simulink model "simrfV2_qpsk"  (R2020b)
settings: Solver=FixedStepDiscrete  StartTime=0.0  StopTime=1600 * SimPars.SampleTime  RelTol=1e-3  EnableMultiTasking=on
PreLoadFcn:
  | SimPars = simrfV2_qpsk_init();
  | load simrfV2_qpsk_patch_antenna.mat;
values from neighbouring files (symbols this model uses):
  lambda = 0.0045423099697    [simrfV2_qpsk_patch_antenna.mat]    (also in simrfV2_qpsk_patch_array_design.m = ps/F0)
  P_isolated = [-26.1777052768 -19.5496256167 -16.1791035724 -14.0467118928 -12.5793492493 -11.5572548786 -10.8860418126 -10.5241336443 -10.4498816598 -10.6370061743 -11.0230573893 -11.4646926094 ... (2701 elements, 37x73)]    [simrfV2_qpsk_patch_antenna.mat]    (also in simrfV2_qpsk_patch_array_design.m = pattern(p, F0))
undefined symbols (not defined in the file or in its folder): phased, physconst, S
libraries: simrfV2util1 x44, simrfV2elements x40, simrfV2junction1 x28, simrfV2systems x8, commrflib2 x3, commdigbbndpm3 x3, dspsigops x3, dspmathops x3, phasedtxrxlib x3, commutil2 x2, commsequence2 x2, commsync2 x2
(part 2 of 2)

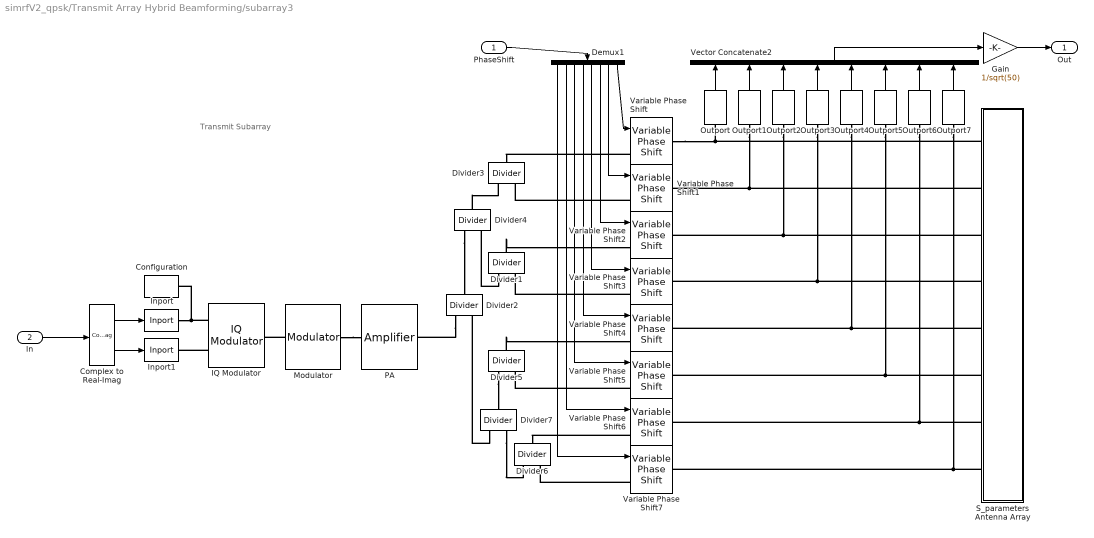
== system simrfV2_qpsk/Transmit Array Hybrid Beamforming/subarray3 ==
  note: Transmit Subarray
  PhaseShift : Inport  OutDataTypeStr=double
  In : Inport  Port=2  OutDataTypeStr=double
      settings: SignalType=complex
  Complex to Real-Imag : ComplexToRealImag
  Configuration : simrfV2util1/Configuration  AutoFreq=off  Tones="[5  66] GHz"  Harmonics=[3 1]  NormalizeCarrierPower=on  SolverType=Auto  UseCCode=on  StepSize=SimPars.SampleTime s  AddNoise=on  defaultRNG=on  Seed=0  Temperature=290.0 K  SolverDelFlag=0  AbsTol=1e-6  RelTol=1e-3  MaxIter=10  ErrorEstimationType=2-norm over all variables  EnableInterpFilter=off  HiddenFIRfilterControllerParam=off  SmallSignalApprox=off  AllSimFreqs=on  SimFreqs=[] Hz  SimFreqsInternal=[]  SamplesPerFrame=SimPars.NumSymsPerFrame * SimPars.SamplesPerSymbol
      settings: SourceProductName=RF Blockset
  Demux1 : Demux  Outputs=8
  Divider{1..7} (7 alike) : simrfV2junction1/Divider  classname=dividers  DataSource=Network-parameters  NumPorts=3  DeviceCirculator=Circulator clockwise  DeviceDivider=Wilkinson power divider  DeviceCoupler=Directional coupler  Paramtype=S-parameters  Sparam=[0 0 1; 1 0 0; 0 1 0]  SparamFreq=1e9 Hz  SparamZ0=50  Phase12=0  Phase33=0  Alpha=0  Coupling=0  Directivity=inf  InsertionLoss=inf  ReturnLoss=inf  InternalGrounding=on  SparamRepresentation=Frequency domain  FitOpt=Share all poles  FitTol=-40
      settings: SourceProductName=RF Blockset
  Gain : Gain  Gain=1/sqrt(50)
  IQ Modulator : simrfV2systems/IQ Modulator  classname=iqmod  Source_linear_gain=Available power gain  linear_gain=8 dB  Poly_Coeffs=[0 1]  LOFreq=5e9 Hz  Zin=50  Zout=50  AddIRFilters=off  AddCSFilter=off  InternalGrounding=on  ForceNextInit=off  NFloor=-168  GainMismatch=0.1 dB  PhaseMismatch=1.2 deg  Isolation=80 dB  AddPhaseNoise=off  PhaseNoiseOffset=1  PhaseNoiseLevel=-Inf  AutoImpulseLengthPN=on  ImpulseLengthPN=1e-10  ImpulseLength_unitPN=s  Source_Poly=Even and odd order  IPType=Output  IP2=21 dBm  IP3=30 dBm  P1dB=inf dBm  Psat=inf dBm  Gcomp=inf dBm  DesignMethodIR=Ideal  ResponseTypeIR=Lowpass  ImplementationIR=LC Tee  ImplementationIdealIR=Constant per carrier  ImplementationRationalIR=Transfer function  UseFilterOrderIR=on  FilterOrderIR=3  PassFreq_lpIR=1  PassFreq_lp_unitIR=GHz  PassFreq_hpIR=2  PassFreq_hp_unitIR=GHz  PassFreq_bpIR=[2 3]  PassFreq_bp_unitIR=GHz  PassFreq_bsIR=[1 4]  PassFreq_bs_unitIR=GHz  PassAttenIR=10*log10(2)  StopFreq_lpIR=2  StopFreq_lp_unitIR=GHz  StopFreq_hpIR=1  StopFreq_hp_unitIR=GHz  StopFreq_bpIR=[1.5 3.5]  StopFreq_bp_unitIR=GHz  StopFreq_bsIR=[2.1 2.9]  StopFreq_bs_unitIR=GHz  StopAttenIR=40  RsrcIR=50  RloadIR=50  AutoImpulseLengthIR=on  ImpulseLengthIR=1e-10  ImpulseLength_unitIR=s  DesignMethodCS=Ideal  ResponseTypeCS=Highpass  ImplementationCS=LC Tee  ImplementationIdealCS=Constant per carrier  ImplementationRationalCS=Transfer function  UseFilterOrderCS=on  FilterOrderCS=3  PassFreq_lpCS=1  PassFreq_lp_unitCS=GHz  PassFreq_hpCS=2  PassFreq_hp_unitCS=GHz  PassFreq_bpCS=[2 3]  PassFreq_bp_unitCS=GHz  PassFreq_bsCS=[1 4]  PassFreq_bs_unitCS=GHz  PassAttenCS=10*log10(2)  StopFreq_lpCS=2  StopFreq_lp_unitCS=GHz  StopFreq_hpCS=1  StopFreq_hp_unitCS=GHz  StopFreq_bpCS=[1.5 3.5]  StopFreq_bp_unitCS=GHz  StopFreq_bsCS=[2.1 2.9]  StopFreq_bs_unitCS=GHz  StopAttenCS=40  RsrcCS=50  RloadCS=50  AutoImpulseLengthCS=on  ImpulseLengthCS=1e-10  ImpulseLength_unitCS=s
      settings: SourceProductName=RF Blockset
  Inport : simrfV2util1/Inport  SimulinkInputSignalType=Power  CarrierFreq=0 Hz  ZS=50  InternalGrounding=on
      settings: SourceProductName=RF Blockset
  Inport1 : simrfV2util1/Inport  SimulinkInputSignalType=Power  CarrierFreq=0 Hz  ZS=50  InternalGrounding=on
      settings: SourceProductName=RF Blockset
  Modulator : simrfV2systems/Modulator  classname=rfmod  Source_linear_gain=Available power gain  linear_gain=-5 dB  Poly_Coeffs=[0 1]  LOFreq=61e9 Hz  Zin=50  Zout=50  AddIRFilter=on  AddCSFilter=on  InternalGrounding=on  ForceNextInit=off  Source_Poly=Even and odd order  IPType=Output  IP2=inf dBm  IP3=inf dBm  P1dB=inf dBm  Psat=inf dBm  Gcomp=inf dBm  NF=6  Isolation=100 dB  AddPhaseNoise=off  PhaseNoiseOffset=1  PhaseNoiseLevel=-Inf  AutoImpulseLengthPN=on  ImpulseLengthPN=1e-10  ImpulseLength_unitPN=s  DesignMethodIR=Ideal  ResponseTypeIR=Lowpass  ImplementationIR=LC Tee  ImplementationIdealIR=Constant per carrier  ImplementationRationalIR=Transfer function  UseFilterOrderIR=on  FilterOrderIR=3  PassFreq_lpIR=10  PassFreq_lp_unitIR=GHz  PassFreq_hpIR=2  PassFreq_hp_unitIR=GHz  PassFreq_bpIR=[2 3]  PassFreq_bp_unitIR=GHz  PassFreq_bsIR=[1 4]  PassFreq_bs_unitIR=GHz  PassAttenIR=10*log10(2)  StopFreq_lpIR=2  StopFreq_lp_unitIR=GHz  StopFreq_hpIR=1  StopFreq_hp_unitIR=GHz  StopFreq_bpIR=[1.5 3.5]  StopFreq_bp_unitIR=GHz  StopFreq_bsIR=[2.1 2.9]  StopFreq_bs_unitIR=GHz  StopAttenIR=40  RsrcIR=50  RloadIR=50  AutoImpulseLengthIR=on  ImpulseLengthIR=1e-10  ImpulseLength_unitIR=s  DesignMethodCS=Ideal  ResponseTypeCS=Highpass  ImplementationCS=LC Tee  ImplementationIdealCS=Constant per carrier  ImplementationRationalCS=Transfer function  UseFilterOrderCS=on  FilterOrderCS=3  PassFreq_lpCS=1  PassFreq_lp_unitCS=GHz  PassFreq_hpCS=60  PassFreq_hp_unitCS=GHz  PassFreq_bpCS=[2 3]  PassFreq_bp_unitCS=GHz  PassFreq_bsCS=[1 4]  PassFreq_bs_unitCS=GHz  PassAttenCS=10*log10(2)  StopFreq_lpCS=2  StopFreq_lp_unitCS=GHz  StopFreq_hpCS=1  StopFreq_hp_unitCS=GHz  StopFreq_bpCS=[1.5 3.5]  StopFreq_bp_unitCS=GHz  StopFreq_bsCS=[2.1 2.9]  StopFreq_bs_unitCS=GHz  StopAttenCS=40  RsrcCS=50  RloadCS=50  AutoImpulseLengthCS=on  ImpulseLengthCS=1e-10  ImpulseLength_unitCS=s
      settings: SourceProductName=RF Blockset
  Outport{,1..7} (8 alike) : simrfV2util1/Outport  SensorType=Ideal voltage  OutputFormat=Complex Baseband  CarrierFreq=SimPars.CarrierFreq Hz  ZL=Inf  InternalGrounding=on  StepSize=1e-6 s  AutoStep=on
      settings: SourceProductName=RF Blockset
  PA : simrfV2elements/Amplifier  classname=amplifier  DataSource=Data file  File=unitygain.s2p  Paramtype=S-parameters  Sparam=[0 0;1 0]  SparamFreq=1e9 Hz  SparamZ0=50  Residues=0  Poles=0  DF={0 0; 1 0}  Source_linear_gain=Available power gain  linear_gain=12 dB  Zin=50  Zout=50  Source_Poly=Odd order  Poly_Coeffs=[0 1]  IPType=Output  IP2=inf dBm  IP3=20 dBm  P1dB=33 dBm  Psat=inf dBm  Gcomp=inf dBm  InternalGrounding=on  SourceFreq=Extracted from data source  PlotFreq=[1e9:1e6:3e9] Hz  PlotType=X-Y plane  YParam1=S(1,1)  YFormat1=Magnitude (decibels)  YParam2=None  YFormat2=Magnitude (decibels)  YOption=Linear  XOption=Linear  SparamRepresentation=Time domain (rationalfit)  FitTol=-40  FitOpt=Fit individually  AutoImpulseLength=on  ImpulseLength=1e-10 s  MagModeling=off  AddNoise=on  NoiseType=Noise figure  NoiseDist=White  NF=3  MinNF=0  Gopt=0  RN=0  CarrierFreq=0 Hz  NoiseAutoImpulseLength=on  NoiseImpulseLength=1e-10 s  SpecifyOpFreq=off  OpFreq=0 Hz
      settings: SourceProductName=RF Blockset
  S_parameters Antenna Array : Subsystem
  Variable Phase Shift{,1..7} (8 alike) : simrfV2elements/Variable Phase Shift  classname=varphase  PhaseShift_unit=deg  SparamZ0=50  InternalGrounding=on
      settings: SourceProductName=RF Blockset
  Vector Concatenate2 : Concatenate  NumInputs=8  Mode=Multidimensional array  ConcatenateDimension=2
  Out : Outport  OutDataTypeStr=double  VectorParamsAs1DForOutWhenUnconnected=off
      settings: SignalType=complex
  wires:
  Outport1/1 -> Vector Concatenate2/2
  Demux1/1 -> Variable Phase Shift7/1
  Demux1/8 -> Variable Phase Shift/1
  Outport6/1 -> Vector Concatenate2/7
  Outport4/1 -> Vector Concatenate2/5
  Complex to Real-Imag/2 -> Inport1/1
  Demux1/7 -> Variable Phase Shift1/1
  Demux1/6 -> Variable Phase Shift2/1
  Demux1/5 -> Variable Phase Shift3/1
  Outport/1 -> Vector Concatenate2/1
  In/1 -> Complex to Real-Imag/1
  Vector Concatenate2/1 -> Gain/1
  Complex to Real-Imag/1 -> Inport/1
  Outport2/1 -> Vector Concatenate2/3
  PhaseShift/1 -> Demux1/1
  Outport5/1 -> Vector Concatenate2/6
  Outport3/1 -> Vector Concatenate2/4
  Demux1/2 -> Variable Phase Shift6/1
  Demux1/3 -> Variable Phase Shift5/1
  Outport7/1 -> Vector Concatenate2/8
  Demux1/4 -> Variable Phase Shift4/1
  Gain/1 -> Out/1
  connections:
  Variable Phase Shift/LConn1 -- Divider3/RConn1
  Outport1/LConn1 -- S_parameters Antenna Array/RConn2 -- Variable Phase Shift1/RConn1
  Divider2/LConn1 -- PA/RConn1
  Outport3/LConn1 -- S_parameters Antenna Array/RConn4 -- Variable Phase Shift3/RConn1
  IQ Modulator/LConn2 -- Inport1/RConn1
  Outport7/LConn1 -- S_parameters Antenna Array/RConn8 -- Variable Phase Shift7/RConn1
  Variable Phase Shift7/LConn1 -- Divider6/LConn2
  Inport/RConn1 -- IQ Modulator/LConn1 -- Configuration/LConn1
  Variable Phase Shift3/LConn1 -- Divider1/LConn2
  Variable Phase Shift/RConn1 -- S_parameters Antenna Array/RConn1 -- Outport/LConn1
  Modulator/RConn1 -- PA/LConn1
  Outport2/LConn1 -- S_parameters Antenna Array/RConn3 -- Variable Phase Shift2/RConn1
  Variable Phase Shift5/LConn1 -- Divider5/LConn2
  Outport6/LConn1 -- S_parameters Antenna Array/RConn7 -- Variable Phase Shift6/RConn1
  Outport5/LConn1 -- S_parameters Antenna Array/RConn6 -- Variable Phase Shift5/RConn1
  Variable Phase Shift6/LConn1 -- Divider6/RConn1
  Divider5/RConn1 -- Variable Phase Shift4/LConn1
  Divider1/RConn1 -- Variable Phase Shift2/LConn1
  Divider4/LConn1 -- Divider2/RConn1
  Divider4/RConn1 -- Divider3/LConn1
  Divider1/LConn1 -- Divider4/LConn2
  Divider5/LConn1 -- Divider7/RConn1
  Divider7/LConn2 -- Divider6/LConn1
  Divider7/LConn1 -- Divider2/LConn2
  Variable Phase Shift1/LConn1 -- Divider3/LConn2
  Modulator/LConn1 -- IQ Modulator/RConn1
  Outport4/LConn1 -- S_parameters Antenna Array/RConn5 -- Variable Phase Shift4/RConn1

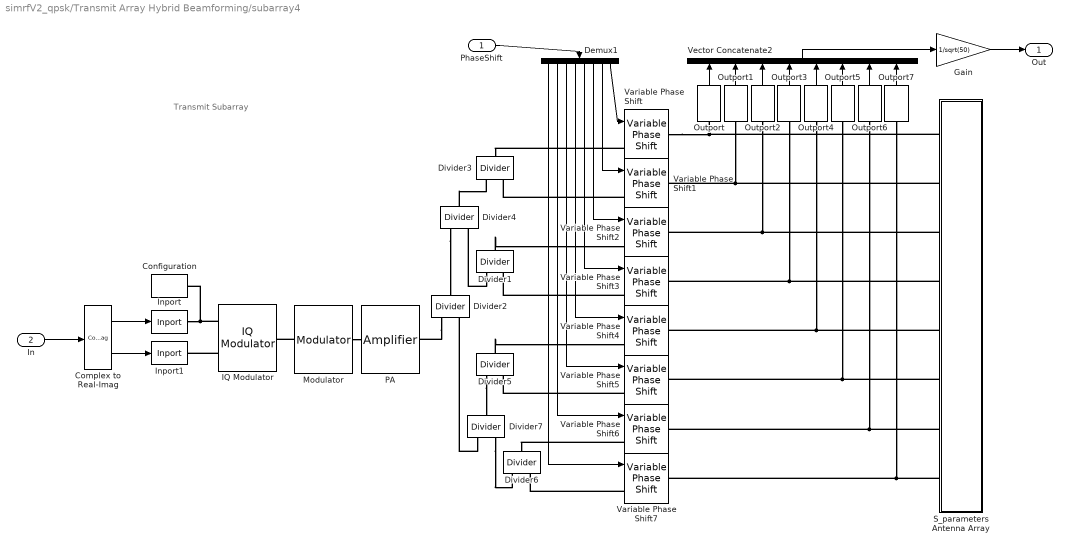
== system simrfV2_qpsk/Transmit Array Hybrid Beamforming/subarray4 ==
  note: Transmit Subarray
  PhaseShift : Inport  OutDataTypeStr=double
  In : Inport  Port=2  OutDataTypeStr=double
      settings: SignalType=complex
  Complex to Real-Imag : ComplexToRealImag
  Configuration : simrfV2util1/Configuration  AutoFreq=off  Tones="[5  66] GHz"  Harmonics=[3 1]  NormalizeCarrierPower=on  SolverType=Auto  UseCCode=on  StepSize=SimPars.SampleTime s  AddNoise=on  defaultRNG=on  Seed=0  Temperature=290.0 K  SolverDelFlag=0  AbsTol=1e-6  RelTol=1e-3  MaxIter=10  ErrorEstimationType=2-norm over all variables  EnableInterpFilter=off  HiddenFIRfilterControllerParam=off  SmallSignalApprox=off  AllSimFreqs=on  SimFreqs=[] Hz  SimFreqsInternal=[]  SamplesPerFrame=SimPars.NumSymsPerFrame * SimPars.SamplesPerSymbol
      settings: SourceProductName=RF Blockset
  Demux1 : Demux  Outputs=8
  Divider{1..7} (7 alike) : simrfV2junction1/Divider  classname=dividers  DataSource=Network-parameters  NumPorts=3  DeviceCirculator=Circulator clockwise  DeviceDivider=Wilkinson power divider  DeviceCoupler=Directional coupler  Paramtype=S-parameters  Sparam=[0 0 1; 1 0 0; 0 1 0]  SparamFreq=1e9 Hz  SparamZ0=50  Phase12=0  Phase33=0  Alpha=0  Coupling=0  Directivity=inf  InsertionLoss=inf  ReturnLoss=inf  InternalGrounding=on  SparamRepresentation=Frequency domain  FitOpt=Share all poles  FitTol=-40
      settings: SourceProductName=RF Blockset
  Gain : Gain  Gain=1/sqrt(50)
  IQ Modulator : simrfV2systems/IQ Modulator  classname=iqmod  Source_linear_gain=Available power gain  linear_gain=8 dB  Poly_Coeffs=[0 1]  LOFreq=5e9 Hz  Zin=50  Zout=50  AddIRFilters=off  AddCSFilter=off  InternalGrounding=on  ForceNextInit=off  NFloor=-168  GainMismatch=0.1 dB  PhaseMismatch=1.2 deg  Isolation=80 dB  AddPhaseNoise=off  PhaseNoiseOffset=1  PhaseNoiseLevel=-Inf  AutoImpulseLengthPN=on  ImpulseLengthPN=1e-10  ImpulseLength_unitPN=s  Source_Poly=Even and odd order  IPType=Output  IP2=21 dBm  IP3=30 dBm  P1dB=inf dBm  Psat=inf dBm  Gcomp=inf dBm  DesignMethodIR=Ideal  ResponseTypeIR=Lowpass  ImplementationIR=LC Tee  ImplementationIdealIR=Constant per carrier  ImplementationRationalIR=Transfer function  UseFilterOrderIR=on  FilterOrderIR=3  PassFreq_lpIR=1  PassFreq_lp_unitIR=GHz  PassFreq_hpIR=2  PassFreq_hp_unitIR=GHz  PassFreq_bpIR=[2 3]  PassFreq_bp_unitIR=GHz  PassFreq_bsIR=[1 4]  PassFreq_bs_unitIR=GHz  PassAttenIR=10*log10(2)  StopFreq_lpIR=2  StopFreq_lp_unitIR=GHz  StopFreq_hpIR=1  StopFreq_hp_unitIR=GHz  StopFreq_bpIR=[1.5 3.5]  StopFreq_bp_unitIR=GHz  StopFreq_bsIR=[2.1 2.9]  StopFreq_bs_unitIR=GHz  StopAttenIR=40  RsrcIR=50  RloadIR=50  AutoImpulseLengthIR=on  ImpulseLengthIR=1e-10  ImpulseLength_unitIR=s  DesignMethodCS=Ideal  ResponseTypeCS=Highpass  ImplementationCS=LC Tee  ImplementationIdealCS=Constant per carrier  ImplementationRationalCS=Transfer function  UseFilterOrderCS=on  FilterOrderCS=3  PassFreq_lpCS=1  PassFreq_lp_unitCS=GHz  PassFreq_hpCS=2  PassFreq_hp_unitCS=GHz  PassFreq_bpCS=[2 3]  PassFreq_bp_unitCS=GHz  PassFreq_bsCS=[1 4]  PassFreq_bs_unitCS=GHz  PassAttenCS=10*log10(2)  StopFreq_lpCS=2  StopFreq_lp_unitCS=GHz  StopFreq_hpCS=1  StopFreq_hp_unitCS=GHz  StopFreq_bpCS=[1.5 3.5]  StopFreq_bp_unitCS=GHz  StopFreq_bsCS=[2.1 2.9]  StopFreq_bs_unitCS=GHz  StopAttenCS=40  RsrcCS=50  RloadCS=50  AutoImpulseLengthCS=on  ImpulseLengthCS=1e-10  ImpulseLength_unitCS=s
      settings: SourceProductName=RF Blockset
  Inport : simrfV2util1/Inport  SimulinkInputSignalType=Power  CarrierFreq=0 Hz  ZS=50  InternalGrounding=on
      settings: SourceProductName=RF Blockset
  Inport1 : simrfV2util1/Inport  SimulinkInputSignalType=Power  CarrierFreq=0 Hz  ZS=50  InternalGrounding=on
      settings: SourceProductName=RF Blockset
  Modulator : simrfV2systems/Modulator  classname=rfmod  Source_linear_gain=Available power gain  linear_gain=-5 dB  Poly_Coeffs=[0 1]  LOFreq=61e9 Hz  Zin=50  Zout=50  AddIRFilter=on  AddCSFilter=on  InternalGrounding=on  ForceNextInit=off  Source_Poly=Even and odd order  IPType=Output  IP2=inf dBm  IP3=inf dBm  P1dB=inf dBm  Psat=inf dBm  Gcomp=inf dBm  NF=6  Isolation=100 dB  AddPhaseNoise=off  PhaseNoiseOffset=1  PhaseNoiseLevel=-Inf  AutoImpulseLengthPN=on  ImpulseLengthPN=1e-10  ImpulseLength_unitPN=s  DesignMethodIR=Ideal  ResponseTypeIR=Lowpass  ImplementationIR=LC Tee  ImplementationIdealIR=Constant per carrier  ImplementationRationalIR=Transfer function  UseFilterOrderIR=on  FilterOrderIR=3  PassFreq_lpIR=10  PassFreq_lp_unitIR=GHz  PassFreq_hpIR=2  PassFreq_hp_unitIR=GHz  PassFreq_bpIR=[2 3]  PassFreq_bp_unitIR=GHz  PassFreq_bsIR=[1 4]  PassFreq_bs_unitIR=GHz  PassAttenIR=10*log10(2)  StopFreq_lpIR=2  StopFreq_lp_unitIR=GHz  StopFreq_hpIR=1  StopFreq_hp_unitIR=GHz  StopFreq_bpIR=[1.5 3.5]  StopFreq_bp_unitIR=GHz  StopFreq_bsIR=[2.1 2.9]  StopFreq_bs_unitIR=GHz  StopAttenIR=40  RsrcIR=50  RloadIR=50  AutoImpulseLengthIR=on  ImpulseLengthIR=1e-10  ImpulseLength_unitIR=s  DesignMethodCS=Ideal  ResponseTypeCS=Highpass  ImplementationCS=LC Tee  ImplementationIdealCS=Constant per carrier  ImplementationRationalCS=Transfer function  UseFilterOrderCS=on  FilterOrderCS=3  PassFreq_lpCS=1  PassFreq_lp_unitCS=GHz  PassFreq_hpCS=60  PassFreq_hp_unitCS=GHz  PassFreq_bpCS=[2 3]  PassFreq_bp_unitCS=GHz  PassFreq_bsCS=[1 4]  PassFreq_bs_unitCS=GHz  PassAttenCS=10*log10(2)  StopFreq_lpCS=2  StopFreq_lp_unitCS=GHz  StopFreq_hpCS=1  StopFreq_hp_unitCS=GHz  StopFreq_bpCS=[1.5 3.5]  StopFreq_bp_unitCS=GHz  StopFreq_bsCS=[2.1 2.9]  StopFreq_bs_unitCS=GHz  StopAttenCS=40  RsrcCS=50  RloadCS=50  AutoImpulseLengthCS=on  ImpulseLengthCS=1e-10  ImpulseLength_unitCS=s
      settings: SourceProductName=RF Blockset
  Outport{,1..7} (8 alike) : simrfV2util1/Outport  SensorType=Ideal voltage  OutputFormat=Complex Baseband  CarrierFreq=SimPars.CarrierFreq Hz  ZL=Inf  InternalGrounding=on  StepSize=1e-6 s  AutoStep=on
      settings: SourceProductName=RF Blockset
  PA : simrfV2elements/Amplifier  classname=amplifier  DataSource=Data file  File=unitygain.s2p  Paramtype=S-parameters  Sparam=[0 0;1 0]  SparamFreq=1e9 Hz  SparamZ0=50  Residues=0  Poles=0  DF={0 0; 1 0}  Source_linear_gain=Available power gain  linear_gain=12 dB  Zin=50  Zout=50  Source_Poly=Odd order  Poly_Coeffs=[0 1]  IPType=Output  IP2=inf dBm  IP3=20 dBm  P1dB=33 dBm  Psat=inf dBm  Gcomp=inf dBm  InternalGrounding=on  SourceFreq=Extracted from data source  PlotFreq=[1e9:1e6:3e9] Hz  PlotType=X-Y plane  YParam1=S(1,1)  YFormat1=Magnitude (decibels)  YParam2=None  YFormat2=Magnitude (decibels)  YOption=Linear  XOption=Linear  SparamRepresentation=Time domain (rationalfit)  FitTol=-40  FitOpt=Fit individually  AutoImpulseLength=on  ImpulseLength=1e-10 s  MagModeling=off  AddNoise=on  NoiseType=Noise figure  NoiseDist=White  NF=3  MinNF=0  Gopt=0  RN=0  CarrierFreq=0 Hz  NoiseAutoImpulseLength=on  NoiseImpulseLength=1e-10 s  SpecifyOpFreq=off  OpFreq=0 Hz
      settings: SourceProductName=RF Blockset
  S_parameters Antenna Array : Subsystem
  Variable Phase Shift{,1..7} (8 alike) : simrfV2elements/Variable Phase Shift  classname=varphase  PhaseShift_unit=deg  SparamZ0=50  InternalGrounding=on
      settings: SourceProductName=RF Blockset
  Vector Concatenate2 : Concatenate  NumInputs=8  Mode=Multidimensional array  ConcatenateDimension=2
  Out : Outport  OutDataTypeStr=double  VectorParamsAs1DForOutWhenUnconnected=off
      settings: SignalType=complex
  wires:
  Outport1/1 -> Vector Concatenate2/2
  Demux1/1 -> Variable Phase Shift7/1
  Demux1/8 -> Variable Phase Shift/1
  Outport6/1 -> Vector Concatenate2/7
  Outport4/1 -> Vector Concatenate2/5
  Complex to Real-Imag/2 -> Inport1/1
  Demux1/7 -> Variable Phase Shift1/1
  Demux1/6 -> Variable Phase Shift2/1
  Demux1/5 -> Variable Phase Shift3/1
  Outport/1 -> Vector Concatenate2/1
  In/1 -> Complex to Real-Imag/1
  Vector Concatenate2/1 -> Gain/1
  Complex to Real-Imag/1 -> Inport/1
  Outport2/1 -> Vector Concatenate2/3
  PhaseShift/1 -> Demux1/1
  Outport5/1 -> Vector Concatenate2/6
  Outport3/1 -> Vector Concatenate2/4
  Demux1/2 -> Variable Phase Shift6/1
  Demux1/3 -> Variable Phase Shift5/1
  Outport7/1 -> Vector Concatenate2/8
  Demux1/4 -> Variable Phase Shift4/1
  Gain/1 -> Out/1
  connections:
  Variable Phase Shift/LConn1 -- Divider3/RConn1
  Outport1/LConn1 -- S_parameters Antenna Array/RConn2 -- Variable Phase Shift1/RConn1
  Divider2/LConn1 -- PA/RConn1
  Outport3/LConn1 -- S_parameters Antenna Array/RConn4 -- Variable Phase Shift3/RConn1
  IQ Modulator/LConn2 -- Inport1/RConn1
  Outport7/LConn1 -- S_parameters Antenna Array/RConn8 -- Variable Phase Shift7/RConn1
  Variable Phase Shift7/LConn1 -- Divider6/LConn2
  Inport/RConn1 -- IQ Modulator/LConn1 -- Configuration/LConn1
  Variable Phase Shift3/LConn1 -- Divider1/LConn2
  Variable Phase Shift/RConn1 -- S_parameters Antenna Array/RConn1 -- Outport/LConn1
  Modulator/RConn1 -- PA/LConn1
  Outport2/LConn1 -- S_parameters Antenna Array/RConn3 -- Variable Phase Shift2/RConn1
  Variable Phase Shift5/LConn1 -- Divider5/LConn2
  Outport6/LConn1 -- S_parameters Antenna Array/RConn7 -- Variable Phase Shift6/RConn1
  Outport5/LConn1 -- S_parameters Antenna Array/RConn6 -- Variable Phase Shift5/RConn1
  Variable Phase Shift6/LConn1 -- Divider6/RConn1
  Divider5/RConn1 -- Variable Phase Shift4/LConn1
  Divider1/RConn1 -- Variable Phase Shift2/LConn1
  Divider4/LConn1 -- Divider2/RConn1
  Divider4/RConn1 -- Divider3/LConn1
  Divider1/LConn1 -- Divider4/LConn2
  Divider5/LConn1 -- Divider7/RConn1
  Divider7/LConn2 -- Divider6/LConn1
  Divider7/LConn1 -- Divider2/LConn2
  Variable Phase Shift1/LConn1 -- Divider3/LConn2
  Modulator/LConn1 -- IQ Modulator/RConn1
  Outport4/LConn1 -- S_parameters Antenna Array/RConn5 -- Variable Phase Shift4/RConn1

== system simrfV2_qpsk/QPSK Receiver/Data Decoding/Barker Code Symbol Generation  ==
  note: Regenerate a QPSK-modulated unipolar Barker code sequence
      | to be compared with the received data
  Constant Barker Code : Constant  Value=SimPars.BarkerCode > 0  VectorParams1D=off  OutDataTypeStr=double
  QPSK Modulator Baseband : commdigbbndpm3/QPSK Modulator Baseband  InType=Bit  Enc=Gray  Ph=pi/4  outDtype=double  outWordLen=16  outUDDataType=sfix(16)  outFracLenMode=Best precision  outFracLen=15  outDataTypeStr=double  outLastDataTypeStr=double
      settings: SourceProductName=Communications Toolbox
  Repeat : dspsigops/Repeat  N=2  InputProcessing=Columns as channels (frame based)  RateOptions=Enforce single-rate processing  ic=0  mode=Unused parameter value
      settings: SourceProductName=DSP System Toolbox
  Out : Outport  VectorParamsAs1DForOutWhenUnconnected=off
  wires:
  Constant Barker Code/1 -> Repeat/1
  Repeat/1 -> QPSK Modulator Baseband/1
  QPSK Modulator Baseband/1 -> Out/1

== system simrfV2_qpsk/QPSK Receiver/Data Decoding/Descrambling ==
  In : Inport
  Descrambler1 : commsequence2/Descrambler  M=2  poly=[1 1 1 0 1]  iniStaSource=Dialog Parameter  ini_sta=[0 0 0 0]  resetViaPort=off
      settings: SourceProductName=Communications Toolbox
  Selector1 : Selector  IndexOptions=Index vector (dialog)  Indices=[2*SimPars.BarkerLength+1:SimPars.NumBitsPerFrame]  OutputSizes=1
  Selector2 : Selector  IndexOptions=Index vector (dialog)  Indices=[1:SimPars.NumMsgBits]  OutputSizes=1
  Out : Outport  VectorParamsAs1DForOutWhenUnconnected=off
  wires:
  In/1 -> Selector1/1
  Selector1/1 -> Descrambler1/1
  Descrambler1/1 -> Selector2/1
  Selector2/1 -> Out/1

== system simrfV2_qpsk/QPSK Receiver/Data Decoding/Phase Ambiguity Correction & Demodulation ==
  note: Phase Ambiguity Resolution
      | and Demodulation
  Phase : Inport
  Data : Inport  Port=2
  Complex Phase Shift : commutil2/Complex Phase Shift
      settings: SourceProductName=Communications Toolbox
  Demodulator Input : ConstellationDiagram
  Gain : Gain  Gain=-1  OutDataTypeStr=Inherit: Same as input
  QPSK Demodulator Baseband : commdigbbndpm3/QPSK Demodulator Baseband  OutType=Bit  DecType=Hard decision  VarSource=Dialog  Variance=1  Dec=Gray  Ph=pi/4  outDtype1=Inherit via internal rule  outDtype2=Inherit via internal rule  derotateFactorWordLen=16  derotateFactorDataTypeStr=Inherit: Same word length as input  derotateFactorLastDataTypeStr=Inherit: Same word length as input
      settings: SourceProductName=Communications Toolbox
  Out : Outport  VectorParamsAs1DForOutWhenUnconnected=off
  wires:
  Phase/1 -> Gain/1
  Complex Phase Shift/1 -> Demodulator Input/1, QPSK Demodulator Baseband/1
  QPSK Demodulator Baseband/1 -> Out/1
  Gain/1 -> Complex Phase Shift/2
  Data/1 -> Complex Phase Shift/1

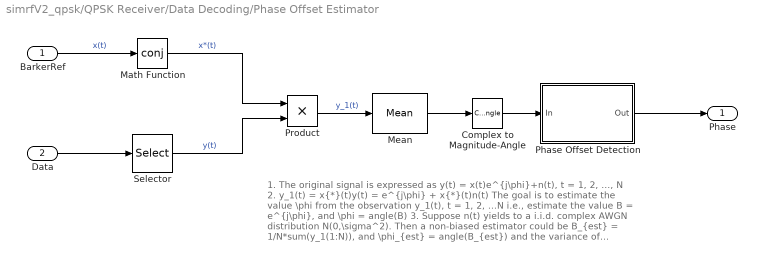
== system simrfV2_qpsk/QPSK Receiver/Data Decoding/Phase Offset Estimator ==
  note: 1. The original signal is expressed as y(t) = x(t)e^{j\phi}+n(t), t = 1, 2, ..., N
      | 2. y_1(t) = x{*}(t)y(t) = e^{j\phi} + x{*}(t)n(t)
      | The goal is to estimate the value \phi from the observation y_1(t), t = 1, 2, ...N
      | i.e., estimate the value B = e^{j\phi}, and \phi = angle(B)
      | 3. Suppose n(t) yields to a i.i.d. complex AWGN distribution N(0,\sigma^2).
      | Then a non-biased estimator could be
      | B_{est} = 1/N*sum(y_1(1:N)), and \phi_{est} = angle(B_{est})
      | and the variance of B_{est} is \sigma^2/N
  BarkerRef : Inport
  Data : Inport  Port=2
  Complex to Magnitude-Angle : ComplexToMagnitudeAngle  Output=Angle
  Math Function : Math  Operator=conj  SignedPower=on  SaturateOnIntegerOverflow=on
  Mean : dspstat3/Mean  run=off  InputProcessing=Columns as channels (frame based)  reset_popup=None  directionMode=Each column  dimension=1  roiEnable=off  roiType=Rectangles  roiPortion=Entire ROI  roiOutput=Individual statistics for each ROI  roiFlag=off  roundingMode=Floor  overflowMode=off  outputDataTypeStr=Inherit: Same as accumulator  outputMin=[]  outputMax=[]  outputLastDataTypeStr=Inherit: Same as accumulator
  Phase Offset Detection : MATLAB Function  TreatAsAtomicUnit=on
  Product : Product  RndMeth=Zero
  Selector : Selector  IndexOptions=Index vector (dialog)  Indices=[1:SimPars.BarkerLength]  OutputSizes=1
  Phase : Outport  VectorParamsAs1DForOutWhenUnconnected=off
  wires:
  Data/1 -> Selector/1
  BarkerRef/1 -> Math Function/1  "x(t)"
  Selector/1 -> Product/2  "y(t)"
  Math Function/1 -> Product/1  "x*(t)"
  Product/1 -> Mean/1  "y_1(t)"
  Mean/1 -> Complex to Magnitude-Angle/1
  Complex to Magnitude-Angle/1 -> Phase Offset Detection/1(In)
  Phase Offset Detection/1(Out) -> Phase/1

== system simrfV2_qpsk/QPSK TX/Bit Generation/Barker Code SS ==
  Barker Code : Constant  Value="SimPars.BarkerCode > 0  % Bipolar to Unipolar Conversion"  VectorParams1D=off
  Data Type Conversion : DataTypeConversion  OutDataTypeStr=double
  Out : Outport  VectorParamsAs1DForOutWhenUnconnected=off
  wires:
  Barker Code/1 -> Data Type Conversion/1
  Data Type Conversion/1 -> Out/1

== system simrfV2_qpsk/QPSK TX/Bit Generation/Message Source ==
  Bernoulli Binary Generator : commrandsrc3/Bernoulli Binary Generator  ProbabilityOfZero=0.5  SeedSource=Parameter  Seed=61  SampleTime=SimPars.BernoulliSampleTime  SamplesPerFrame=SimPars.BernoulliFrameBits  OutputDataType=double  SimulateUsing=Code generation
      settings: SourceProductName=Communications Toolbox
  Matrix Concatenate : Concatenate  Mode=Multidimensional array
  Message Generator : MATLAB Function  TreatAsAtomicUnit=on
  Out : Outport  VectorParamsAs1DForOutWhenUnconnected=off
  wires:
  Message Generator/1(msg) -> Matrix Concatenate/1
  Bernoulli Binary Generator/1 -> Matrix Concatenate/2
  Matrix Concatenate/1 -> Out/1

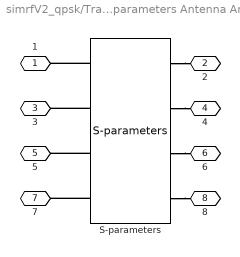
== system simrfV2_qpsk/Transmit Array Hybrid Beamforming/subarray1/S_parameters Antenna Array ==
  S-parameters : simrfV2elements/S-parameters  classname=sparam_element  DataSource=Network-parameters  File=unitygain.s2p  Paramtype=S-parameters  Sparam=Spars.Parameters  SparamFreq=Spars.Frequencies Hz  SparamZ0=50  Residues=0  Poles=0  DF={0 0; 1 0}  FitOpt=Share all poles  FitTol=-40  SourceFreq=Extracted from data source  PlotFreq=[1e9:1e6:3e9] Hz  PlotType=X-Y plane  YParam1=S(1,1)  YFormat1=Magnitude (decibels)  YParam2=S(1,2)  YFormat2=Magnitude (decibels)  YOption=Linear  XOption=Linear  AddNoise=on  InternalGrounding=on  SparamRepresentation=Frequency domain  AutoImpulseLength=on  ImpulseLength=1e-10 s  MagModeling=off  CacheLevel=0
      settings: SourceProductName=RF Blockset
  1 : PMIOPort  Side=Right
  2 : PMIOPort  Port=2  Side=Right
  3 : PMIOPort  Port=3  Side=Right
  4 : PMIOPort  Port=4  Side=Right
  5 : PMIOPort  Port=5  Side=Right
  6 : PMIOPort  Port=6  Side=Right
  7 : PMIOPort  Port=7  Side=Right
  8 : PMIOPort  Port=8  Side=Right
  connections:
  S-parameters/RConn1 -- 2/RConn1
  S-parameters/LConn4 -- 7/RConn1
  S-parameters/LConn3 -- 5/RConn1
  S-parameters/RConn3 -- 6/RConn1
  S-parameters/LConn2 -- 3/RConn1
  S-parameters/RConn4 -- 8/RConn1
  S-parameters/RConn2 -- 4/RConn1
  S-parameters/LConn1 -- 1/RConn1

== system simrfV2_qpsk/Transmit Array Hybrid Beamforming/subarray2/S_parameters Antenna Array ==
  S-parameters : simrfV2elements/S-parameters  classname=sparam_element  DataSource=Network-parameters  File=unitygain.s2p  Paramtype=S-parameters  Sparam=Spars.Parameters  SparamFreq=Spars.Frequencies Hz  SparamZ0=50  Residues=0  Poles=0  DF={0 0; 1 0}  FitOpt=Share all poles  FitTol=-40  SourceFreq=Extracted from data source  PlotFreq=[1e9:1e6:3e9] Hz  PlotType=X-Y plane  YParam1=S(1,1)  YFormat1=Magnitude (decibels)  YParam2=S(1,2)  YFormat2=Magnitude (decibels)  YOption=Linear  XOption=Linear  AddNoise=on  InternalGrounding=on  SparamRepresentation=Frequency domain  AutoImpulseLength=on  ImpulseLength=1e-10 s  MagModeling=off  CacheLevel=0
      settings: SourceProductName=RF Blockset
  1 : PMIOPort  Side=Right
  2 : PMIOPort  Port=2  Side=Right
  3 : PMIOPort  Port=3  Side=Right
  4 : PMIOPort  Port=4  Side=Right
  5 : PMIOPort  Port=5  Side=Right
  6 : PMIOPort  Port=6  Side=Right
  7 : PMIOPort  Port=7  Side=Right
  8 : PMIOPort  Port=8  Side=Right
  connections:
  S-parameters/RConn1 -- 2/RConn1
  S-parameters/LConn4 -- 7/RConn1
  S-parameters/LConn3 -- 5/RConn1
  S-parameters/RConn3 -- 6/RConn1
  S-parameters/LConn2 -- 3/RConn1
  S-parameters/RConn4 -- 8/RConn1
  S-parameters/RConn2 -- 4/RConn1
  S-parameters/LConn1 -- 1/RConn1

== system simrfV2_qpsk/Transmit Array Hybrid Beamforming/subarray3/S_parameters Antenna Array ==
  S-parameters : simrfV2elements/S-parameters  classname=sparam_element  DataSource=Network-parameters  File=unitygain.s2p  Paramtype=S-parameters  Sparam=Spars.Parameters  SparamFreq=Spars.Frequencies Hz  SparamZ0=50  Residues=0  Poles=0  DF={0 0; 1 0}  FitOpt=Share all poles  FitTol=-40  SourceFreq=Extracted from data source  PlotFreq=[1e9:1e6:3e9] Hz  PlotType=X-Y plane  YParam1=S(1,1)  YFormat1=Magnitude (decibels)  YParam2=S(1,2)  YFormat2=Magnitude (decibels)  YOption=Linear  XOption=Linear  AddNoise=on  InternalGrounding=on  SparamRepresentation=Frequency domain  AutoImpulseLength=on  ImpulseLength=1e-10 s  MagModeling=off  CacheLevel=0
      settings: SourceProductName=RF Blockset
  1 : PMIOPort  Side=Right
  2 : PMIOPort  Port=2  Side=Right
  3 : PMIOPort  Port=3  Side=Right
  4 : PMIOPort  Port=4  Side=Right
  5 : PMIOPort  Port=5  Side=Right
  6 : PMIOPort  Port=6  Side=Right
  7 : PMIOPort  Port=7  Side=Right
  8 : PMIOPort  Port=8  Side=Right
  connections:
  S-parameters/RConn1 -- 2/RConn1
  S-parameters/LConn4 -- 7/RConn1
  S-parameters/LConn3 -- 5/RConn1
  S-parameters/RConn3 -- 6/RConn1
  S-parameters/LConn2 -- 3/RConn1
  S-parameters/RConn4 -- 8/RConn1
  S-parameters/RConn2 -- 4/RConn1
  S-parameters/LConn1 -- 1/RConn1

== system simrfV2_qpsk/Transmit Array Hybrid Beamforming/subarray4/S_parameters Antenna Array ==
  S-parameters : simrfV2elements/S-parameters  classname=sparam_element  DataSource=Network-parameters  File=unitygain.s2p  Paramtype=S-parameters  Sparam=Spars.Parameters  SparamFreq=Spars.Frequencies Hz  SparamZ0=50  Residues=0  Poles=0  DF={0 0; 1 0}  FitOpt=Share all poles  FitTol=-40  SourceFreq=Extracted from data source  PlotFreq=[1e9:1e6:3e9] Hz  PlotType=X-Y plane  YParam1=S(1,1)  YFormat1=Magnitude (decibels)  YParam2=S(1,2)  YFormat2=Magnitude (decibels)  YOption=Linear  XOption=Linear  AddNoise=on  InternalGrounding=on  SparamRepresentation=Frequency domain  AutoImpulseLength=on  ImpulseLength=1e-10 s  MagModeling=off  CacheLevel=0
      settings: SourceProductName=RF Blockset
  1 : PMIOPort  Side=Right
  2 : PMIOPort  Port=2  Side=Right
  3 : PMIOPort  Port=3  Side=Right
  4 : PMIOPort  Port=4  Side=Right
  5 : PMIOPort  Port=5  Side=Right
  6 : PMIOPort  Port=6  Side=Right
  7 : PMIOPort  Port=7  Side=Right
  8 : PMIOPort  Port=8  Side=Right
  connections:
  S-parameters/RConn1 -- 2/RConn1
  S-parameters/LConn4 -- 7/RConn1
  S-parameters/LConn3 -- 5/RConn1
  S-parameters/RConn3 -- 6/RConn1
  S-parameters/LConn2 -- 3/RConn1
  S-parameters/RConn4 -- 8/RConn1
  S-parameters/RConn2 -- 4/RConn1
  S-parameters/LConn1 -- 1/RConn1

== matlab function simrfV2_qpsk/QPSK TX/Bit Generation/Message Source/Message Generator ==
  data: msg output
function msg = genMsg
%#codegen
persistent msgStrSet count;
if isempty(msgStrSet)
    count = 0;
    msgStrSet = [
        'Hello world 000';                                              ...
        'Hello world 001';                                              ...
        'Hello world 002';                                              ...
        'Hello world 003';                                              ...
        'Hello world 004';                                              ...
        'Hello world 005';                                              ...
        'Hello world 006';                                              ...
        'Hello world 007';                                              ...
        'Hello world 008';                                              ...
        'Hello world 009';                                              ...
        'Hello world 010';                                              ...
        'Hello world 011';                                              ...
        'Hello world 012';                                              ...
        'Hello world 013';                                              ...
        'Hello world 014';                                              ...
        'Hello world 015';                                              ...
        'Hello world 016';                                              ...
        'Hello world 017';                                              ...
        'Hello world 018';                                              ...
        'Hello world 019';                                              ...
        'Hello world 020';                                              ...
        'Hello world 021';                                              ...
        'Hello world 022';                                              ...
        'Hello world 023';                                              ...
        'Hello world 024';                                              ...
        'Hello world 025';                                              ...
        'Hello world 026';                                              ...
        'Hello world 027';                                              ...
        'Hello world 028';                                              ...
        'Hello world 029';                                              ...
        'Hello world 030';                                              ...
        'Hello world 031';                                              ...
        'Hello world 032';                                              ...
        'Hello world 033';                                              ...
        'Hello world 034';                                              ...
        'Hello world 035';                                              ...
        'Hello world 036';                                              ...
        'Hello world 037';                                              ...
        'Hello world 038';                                              ...
        'Hello world 039';                                              ...
        'Hello world 040';                                              ...
        'Hello world 041';                                              ...
        'Hello world 042';                                              ...
        'Hello world 043';                                              ...
        'Hello world 044';                                              ...
        'Hello world 045';                                              ...
        'Hello world 046';                                              ...
        'Hello world 047';                                              ...
        'Hello world 048';                                              ...
        'Hello world 049';                                              ...
        'Hello world 050';                                              ...
        'Hello world 051';                                              ...
        'Hello world 052';                                              ...
        'Hello world 053';                                              ...
        'Hello world 054';                                              ...
        'Hello world 055';                                              ...
        'Hello world 056';                                              ...
        'Hello world 057';                                              ...
        'Hello world 058';                                              ...
        'Hello world 059';                                              ...
        'Hello world 060';                                              ...
        'Hello world 061';                                              ...
        'Hello world 062';                                              ...
        'Hello world 063';                                              ...
        'Hello world 064';                                              ...
        'Hello world 065';                                              ...
        'Hello world 066';                                              ...
        'Hello world 067';                                              ...
        'Hello world 068';                                              ...
        'Hello world 069';                                              ...
        'Hello world 070';                                              ...
        'Hello world 071';                                              ...
        'Hello world 072';                                              ...
        'Hello world 073';                                              ...
        'Hello world 074';                                              ...
        'Hello world 075';                                              ...
        'Hello world 076';                                              ...
        'Hello world 077';                                              ...
        'Hello world 078';                                              ...
        'Hello world 079';                                              ...
        'Hello world 080';                                              ...
        'Hello world 081';                                              ...
        'Hello world 082';                                              ...
        'Hello world 083';                                              ...
        'Hello world 084';                                              ...
        'Hello world 085';                                              ...
        'Hello world 086';                                              ...
        'Hello world 087';                                              ...
        'Hello world 088';                                              ...
        'Hello world 089';                                              ...
        'Hello world 090';                                              ...
        'Hello world 091';                                              ...
        'Hello world 092';                                              ...
        'Hello world 093';                                              ...
        'Hello world 094';                                              ...
        'Hello world 095';                                              ...
        'Hello world 096';                                              ...
        'Hello world 097';                                              ...
        'Hello world 098';                                              ...
        'Hello world 099'];
end

msgStr = msgStrSet(count+1,:);
msgBin = de2bi(int8(msgStr),7,'left-msb');
msg = reshape(double(msgBin).',105,1);
count = mod(count+1,100);

== matlab function simrfV2_qpsk/QPSK Receiver/Data Decoding/Phase Offset Estimator/Phase Offset Detection ==
  data: In input; Out output
function Out = phasedecision(In)
% Map the estimated phase to one of -pi, -pi/2, 0, pi/2,  
%#codegen
Out = round(In.*2./pi)./2.*pi;
% The above processing is equivalent to the following processing using
% if/else statements
%
% if In<pi/4 && In>-pi/4
%     Out = 0;
% elseif In>=pi/4 && In<pi*3/4
%     Out = pi/2;
% elseif In>=pi*3/4 || In<=-pi*3/4
%     Out = -pi;
% else
%     Out = -pi/2;
% end
